simulink library "sensors_T2_design_lib"  (R2023b)
settings: Solver=ode45  StartTime=0.0  StopTime=10.0  RelTol=1e-3  EnableMultiTasking=on
undefined symbols (not defined in the file or in its folder): POS_hi, POS_lo, Timestep
libraries: NoiseModel_lib x16, simulink_extras x3, TransportDelay_lib x1, simulink x1
settings Model: Creator=amurch  LastModifiedBy=suvo
settings SolverCC: AlgebraicLoopSolver=TrustRegion
settings DataIOCC: LimitDataPoints=on  SaveFormat=Array  SignalLoggingSaveFormat=ModelDataLogs  ReturnWorkspaceOutputs=off
settings OptimizationCC: ExpressionDepthLimit=2147483647  LifeSpan=inf
settings DebuggingCC: UnderspecifiedInitializationDetection=Classic  MergeDetectMultiDrivingBlocksExec=none  SolverPrmCheckMsg=warning  FcnCallInpInsideContextMsg=warning  UnconnectedInputMsg=warning  UnconnectedOutputMsg=warning  UnconnectedLineMsg=warning  StateNameClashWarn=warning  SFUnexpectedBacktrackingDiag=warning  SFNoUnconditionalDefaultTransitionDiag=warning  SFExecutionAtInitializationDiag=none  ArithmeticOperatorsInVariantConditions=warning
settings HardwareCC: ProdBitPerPointer=32  ProdBitPerSizeT=32  ProdBitPerPtrDiffT=32  ProdLargestAtomicFloat=None  ProdIntDivRoundTo=Undefined  ProdEndianess=Unspecified  ProdWordSize=32  ProdHWDeviceType=32-bit Generic
settings ModelReferenceCC: PropagateSignalLabelsOutOfModel=off
settings SFSimCC: SimUseLocalCustomCode=off  CustomCodeUndefinedFunction=UseInterfaceOnly
settings RTWCC: RTWUseLocalCustomCode=off
settings CodeAppCC: StateflowObjectComments=on
settings GRTTargetCC: TargetLangStandard=C89/C90 (ANSI)  CombineOutputUpdateFcns=off  GRTInterface=on
settings ConfigComp: CovMetricSettings=dw  CovSaveCumulativeToWorkspaceVar=on  CovSaveSingleToWorkspaceVar=on

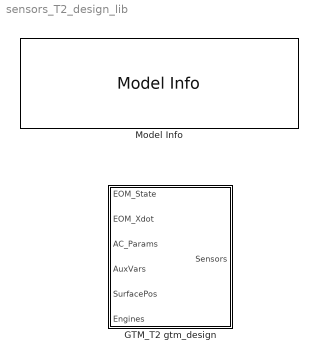
== system sensors_T2_design_lib ==
  GTM_T2 gtm_design : Subsystem
  Model Info : simulink/Model-Wide Utilities/Model Info  Frame=on  DisplayStringWithTags=|  HorizontalTextAlignment=Center  LeftAlignmentValue=0.5
      | Sensor Model Library
      | %<ModelVersion>
      | Las modified by %<LastModifiedBy> on %<LastModificationDate>

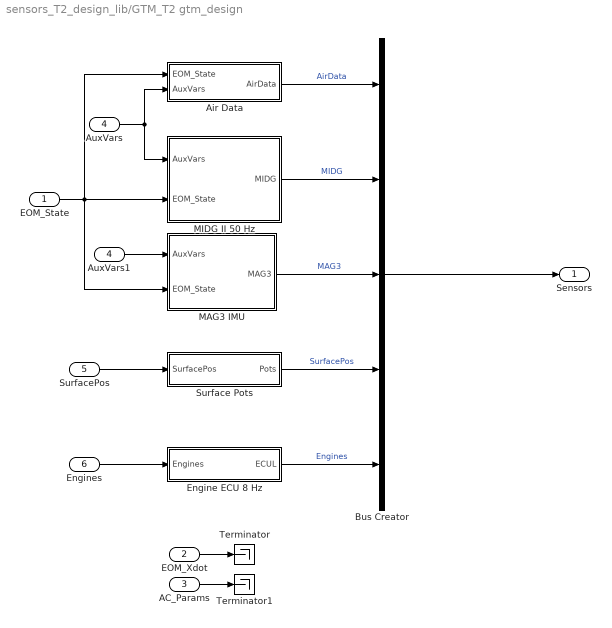
== system sensors_T2_design_lib/GTM_T2 gtm_design ==
  EOM_State : Inport
  EOM_Xdot : Inport  Port=2
  AC_Params : Inport  Port=3
  AuxVars : Inport  Port=4
  SurfacePos : Inport  Port=5
  Engines : Inport  Port=6
  Air Data : Subsystem
  AuxVars1 : InportShadow  Port=4
  Bus Creator : BusCreator  Inputs=5
  Engine ECU 8 Hz : Subsystem  SystemSampleTime=round(1/Timestep/8)*Timestep
  MAG3 IMU : Subsystem
  MIDG II 50 Hz : Subsystem  SystemSampleTime=round(1/Timestep/50)*Timestep
  Surface Pots : Subsystem
  Terminator : Terminator
  Terminator1 : Terminator
  Sensors : Outport
  wires:
  AuxVars1/1 -> MAG3 IMU/1(AuxVars)
  EOM_State/1 -> Air Data/1(EOM_State), MIDG II 50 Hz/2(EOM_State), MAG3 IMU/2(EOM_State)
  AuxVars/1 -> MIDG II 50 Hz/1(AuxVars), Air Data/2(AuxVars)
  SurfacePos/1 -> Surface Pots/1(SurfacePos)
  Engines/1 -> Engine ECU 8 Hz/1(Engines)
  MAG3 IMU/1(MAG3) -> Bus Creator/3  "MAG3"
  Engine ECU 8 Hz/1(ECUL) -> Bus Creator/5  "Engines"
  Surface Pots/1(Pots) -> Bus Creator/4  "SurfacePos"
  MIDG II 50 Hz/1(MIDG) -> Bus Creator/2  "MIDG"
  Air Data/1(AirData) -> Bus Creator/1  "AirData"
  Bus Creator/1 -> Sensors/1
  EOM_Xdot/1 -> Terminator/1
  AC_Params/1 -> Terminator1/1

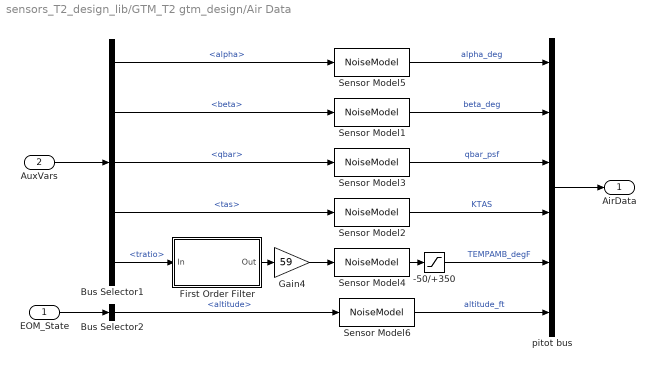
== system sensors_T2_design_lib/GTM_T2 gtm_design/Air Data ==
  EOM_State : Inport
  AuxVars : Inport  Port=2
  -50/+350 : Saturate  UpperLimit=350  LowerLimit=-50
  Bus Selector1 : BusSelector  OutputSignals=alpha,beta,qbar,tas,tratio
  Bus Selector2 : BusSelector  OutputSignals=altitude
  First Order Filter : Subsystem  mask(first order filter){tau=6}
      mask help:
      | __1__
      |  tau s+1
      |
      | First order filter  transfer function
      | with integrator IC = input  at time=0
      | If tau < Simulation Timestep, input is passed through unchanged
      | Simulation timestep must be a variable in the model/base workspace named
      | "Timestep"
      mask Help:
      | This block models a first order filter with the initial condition
      | on the integrator set to the steady state value for constant input.
      | time constant is an input
      mask Display: fprintf('  1\n--------------\n %2.1g s + 1', tau)
  Gain4 : Gain  Gain=59
  Sensor Model1 : NoiseModel_lib/NoiseModel  SystemSampleTime=-1  noise_on=SensorNoise.On  sigma=SensorNoise.beta.Std  seed=878224  bias=SensorNoise.beta.Bias  scf=SensorNoise.beta.Scf
  Sensor Model2 : NoiseModel_lib/NoiseModel  SystemSampleTime=-1  noise_on=SensorNoise.On  sigma=SensorNoise.KTAS.Std  seed=878654  bias=SensorNoise.KTAS.Bias  scf=SensorNoise.KTAS.Scf
  Sensor Model3 : NoiseModel_lib/NoiseModel  SystemSampleTime=-1  noise_on=SensorNoise.On  sigma=SensorNoise.dyn_press.Std  seed=848234  bias=SensorNoise.dyn_press.Bias  scf=SensorNoise.dyn_press.Scf
  Sensor Model4 : NoiseModel_lib/NoiseModel  SystemSampleTime=-1  noise_on=SensorNoise.On  sigma=SensorNoise.tempamb.Std  seed=878634  bias=SensorNoise.tempamb.Bias  scf=SensorNoise.tempamb.Scf
  Sensor Model5 : NoiseModel_lib/NoiseModel  SystemSampleTime=-1  noise_on=SensorNoise.On  sigma=SensorNoise.alpha.Std  seed=278234  bias=SensorNoise.alpha.Bias  scf=SensorNoise.alpha.Scf
  Sensor Model6 : NoiseModel_lib/NoiseModel  SystemSampleTime=-1  noise_on=SensorNoise.On  sigma=SensorNoise.baro_alt.Std  seed=878654  bias=SensorNoise.baro_alt.Bias  scf=SensorNoise.baro_alt.Scf
  pitot bus : BusCreator  Inputs=6
  AirData : Outport
  wires:
  EOM_State/1 -> Bus Selector2/1
  Sensor Model6/1 -> pitot bus/6  "altitude_ft"
  Bus Selector2/1 -> Sensor Model6/1  "<altitude>"
  AuxVars/1 -> Bus Selector1/1
  Sensor Model2/1 -> pitot bus/4  "KTAS"
  Bus Selector1/4 -> Sensor Model2/1  "<tas>"
  Sensor Model1/1 -> pitot bus/2  "beta_deg"
  Sensor Model5/1 -> pitot bus/1  "alpha_deg"
  Bus Selector1/2 -> Sensor Model1/1  "<beta>"
  Bus Selector1/1 -> Sensor Model5/1  "<alpha>"
  First Order Filter/1(Out) -> Gain4/1
  -50/+350/1 -> pitot bus/5  "TEMPAMB_degF"
  Sensor Model4/1 -> -50/+350/1
  Gain4/1 -> Sensor Model4/1
  pitot bus/1 -> AirData/1
  Bus Selector1/3 -> Sensor Model3/1  "<qbar>"
  Sensor Model3/1 -> pitot bus/3  "qbar_psf"
  Bus Selector1/5 -> First Order Filter/1(In)  "<tratio>"

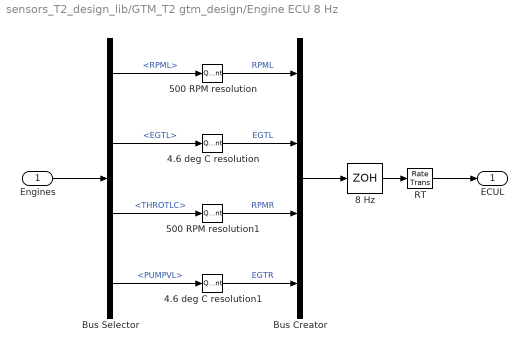
== system sensors_T2_design_lib/GTM_T2 gtm_design/Engine ECU 8 Hz ==
  Engines : Inport
  4.6 deg C resolution : Quantizer  QuantizationInterval=4.6
  4.6 deg C resolution1 : Quantizer  QuantizationInterval=4.6
  500 RPM resolution : Quantizer  QuantizationInterval=500
  500 RPM resolution1 : Quantizer  QuantizationInterval=500
  8 Hz : ZeroOrderHold  SampleTime=round(1/Timestep/8)*Timestep
  Bus Creator : BusCreator  Inputs=4
  Bus Selector : BusSelector  OutputSignals=RPML,EGTL,THROTLC,PUMPVL
  RT : RateTransition
  ECUL : Outport
  wires:
  4.6 deg C resolution1/1 -> Bus Creator/4  "EGTR"
  Bus Selector/4 -> 4.6 deg C resolution1/1  "<PUMPVL>"
  500 RPM resolution1/1 -> Bus Creator/3  "RPMR"
  Bus Selector/3 -> 500 RPM resolution1/1  "<THROTLC>"
  Engines/1 -> Bus Selector/1
  4.6 deg C resolution/1 -> Bus Creator/2  "EGTL"
  500 RPM resolution/1 -> Bus Creator/1  "RPML"
  Bus Selector/1 -> 500 RPM resolution/1  "<RPML>"
  RT/1 -> ECUL/1
  Bus Creator/1 -> 8 Hz/1
  8 Hz/1 -> RT/1
  Bus Selector/2 -> 4.6 deg C resolution/1  "<EGTL>"

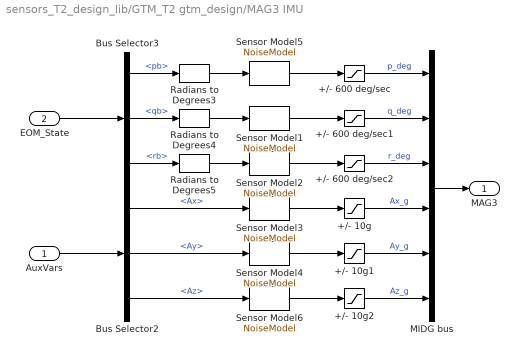
== system sensors_T2_design_lib/GTM_T2 gtm_design/MAG3 IMU ==
  AuxVars : Inport
  EOM_State : Inport  Port=2
  +/- 10g : Saturate  UpperLimit=10  LowerLimit=-10
  +/- 10g1 : Saturate  UpperLimit=10  LowerLimit=-10
  +/- 10g2 : Saturate  UpperLimit=10  LowerLimit=-10
  +/- 600 deg/sec : Saturate  UpperLimit=600  LowerLimit=-600
  +/- 600 deg/sec1 : Saturate  UpperLimit=600  LowerLimit=-600
  +/- 600 deg/sec2 : Saturate  UpperLimit=600  LowerLimit=-600
  Bus Selector2 : BusSelector  OutputSignals=Ax,Ay,Az
  Bus Selector3 : BusSelector  OutputSignals=pb,qb,rb
  MIDG bus : BusCreator  Inputs=6
  Radians to Degrees3 : simulink_extras/Transformations/Radians to Degrees  SystemSampleTime=-1
  Radians to Degrees4 : simulink_extras/Transformations/Radians to Degrees  SystemSampleTime=-1
  Radians to Degrees5 : simulink_extras/Transformations/Radians to Degrees  SystemSampleTime=-1
  Sensor Model1 : NoiseModel_lib/NoiseModel  SystemSampleTime=-1  noise_on=SensorNoise.On  sigma=SensorNoise.MAG3.qdeg.Std  seed=871234  bias=SensorNoise.MAG3.qdeg.Bias  scf=SensorNoise.MAG3.qdeg.Scf
  Sensor Model2 : NoiseModel_lib/NoiseModel  SystemSampleTime=-1  noise_on=SensorNoise.On  sigma=SensorNoise.MAG3.rdeg.Std  seed=878134  bias=SensorNoise.MAG3.rdeg.Bias  scf=SensorNoise.MAG3.rdeg.Scf
  Sensor Model3 : NoiseModel_lib/NoiseModel  SystemSampleTime=-1  noise_on=SensorNoise.On  sigma=SensorNoise.MAG3.nxbody.Std  seed=878234  bias=SensorNoise.MAG3.nxbody.Bias  scf=SensorNoise.MAG3.nxbody.Scf
  Sensor Model4 : NoiseModel_lib/NoiseModel  SystemSampleTime=-1  noise_on=SensorNoise.On  sigma=SensorNoise.MAG3.nybody.Std  seed=8782345  bias=SensorNoise.MAG3.nybody.Bias  scf=SensorNoise.MAG3.nybody.Scf
  Sensor Model5 : NoiseModel_lib/NoiseModel  SystemSampleTime=-1  noise_on=SensorNoise.On  sigma=SensorNoise.MAG3.pdeg.Std  seed=878233  bias=SensorNoise.MAG3.pdeg.Bias  scf=SensorNoise.MAG3.pdeg.Scf
  Sensor Model6 : NoiseModel_lib/NoiseModel  SystemSampleTime=-1  noise_on=SensorNoise.On  sigma=SensorNoise.MAG3.nzbody.Std  seed=878236  bias=SensorNoise.MAG3.nzbody.Bias  scf=SensorNoise.MAG3.nzbody.Scf
  MAG3 : Outport
  wires:
  MIDG bus/1 -> MAG3/1
  AuxVars/1 -> Bus Selector2/1
  Sensor Model5/1 -> +/- 600 deg/sec/1
  Sensor Model6/1 -> +/- 10g2/1
  Sensor Model4/1 -> +/- 10g1/1
  Sensor Model3/1 -> +/- 10g/1
  Sensor Model2/1 -> +/- 600 deg/sec2/1
  Sensor Model1/1 -> +/- 600 deg/sec1/1
  Radians to Degrees5/1 -> Sensor Model2/1
  Radians to Degrees4/1 -> Sensor Model1/1
  Radians to Degrees3/1 -> Sensor Model5/1
  Bus Selector2/3 -> Sensor Model6/1  "<Az>"
  Bus Selector2/2 -> Sensor Model4/1  "<Ay>"
  Bus Selector2/1 -> Sensor Model3/1  "<Ax>"
  Bus Selector3/3 -> Radians to Degrees5/1  "<rb>"
  Bus Selector3/2 -> Radians to Degrees4/1  "<qb>"
  Bus Selector3/1 -> Radians to Degrees3/1  "<pb>"
  EOM_State/1 -> Bus Selector3/1
  +/- 600 deg/sec/1 -> MIDG bus/1  "p_deg"
  +/- 600 deg/sec1/1 -> MIDG bus/2  "q_deg"
  +/- 600 deg/sec2/1 -> MIDG bus/3  "r_deg"
  +/- 10g/1 -> MIDG bus/4  "Ax_g"
  +/- 10g1/1 -> MIDG bus/5  "Ay_g"
  +/- 10g2/1 -> MIDG bus/6  "Az_g"

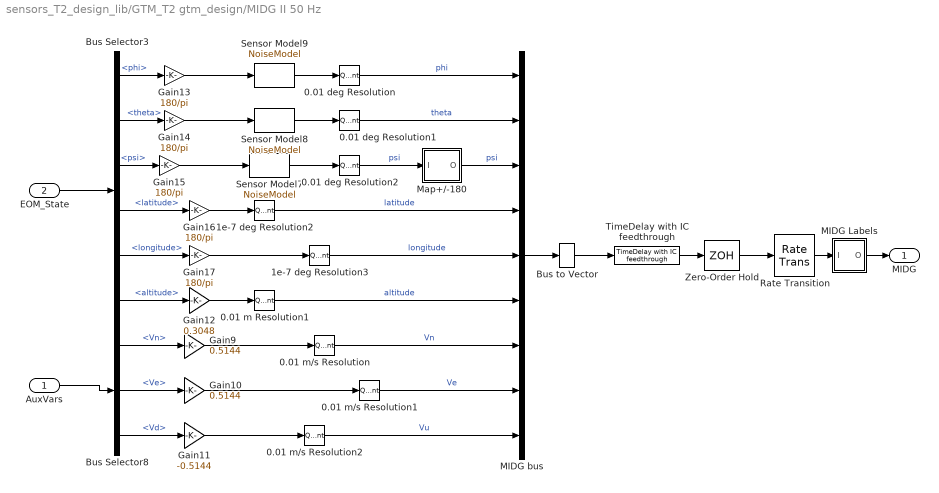
== system sensors_T2_design_lib/GTM_T2 gtm_design/MIDG II 50 Hz ==
  AuxVars : Inport
  EOM_State : Inport  Port=2
  0.01 deg Resolution : Quantizer  QuantizationInterval=0.01
  0.01 deg Resolution1 : Quantizer  QuantizationInterval=0.01
  0.01 deg Resolution2 : Quantizer  QuantizationInterval=0.01
  0.01 m Resolution1 : Quantizer  QuantizationInterval=0.01
  0.01 m/s Resolution : Quantizer  QuantizationInterval=0.01
  0.01 m/s Resolution1 : Quantizer  QuantizationInterval=0.01
  0.01 m/s Resolution2 : Quantizer  QuantizationInterval=0.01
  1e-7 deg Resolution2 : Quantizer  QuantizationInterval=1e-7
  1e-7 deg Resolution3 : Quantizer  QuantizationInterval=1e-7
  Bus Selector3 : BusSelector  OutputSignals=phi,theta,psi,latitude,longitude,altitude
  Bus Selector8 : BusSelector  OutputSignals=Vn,Ve,Vd
  Bus to Vector : BusToVector
  Gain10 : Gain  Gain=0.5144
  Gain11 : Gain  Gain=-0.5144
  Gain12 : Gain  Gain=0.3048
  Gain{13..17} (5 alike) : Gain  Gain=180/pi
  Gain9 : Gain  Gain=0.5144
  MIDG Labels : Subsystem
  MIDG bus : BusCreator  Inputs=9
  Map+/-180 : Subsystem
  Rate Transition : RateTransition
  Sensor Model7 : NoiseModel_lib/NoiseModel  SystemSampleTime=-1  noise_on=SensorNoise.On  sigma=SensorNoise.MIDG.psi.Std  seed=878232  bias=SensorNoise.MIDG.psi.Bias  scf=SensorNoise.MIDG.psi.Scf
  Sensor Model8 : NoiseModel_lib/NoiseModel  SystemSampleTime=-1  noise_on=SensorNoise.On  sigma=SensorNoise.MIDG.theta.Std  seed=878231  bias=SensorNoise.MIDG.theta.Bias  scf=SensorNoise.MIDG.theta.Scf
  Sensor Model9 : NoiseModel_lib/NoiseModel  SystemSampleTime=-1  noise_on=SensorNoise.On  sigma=SensorNoise.MIDG.phi.Std  seed=878230  bias=SensorNoise.MIDG.phi.Bias  scf=SensorNoise.MIDG.phi.Scf
  TimeDelay with IC feedthrough : TransportDelay_lib/TimeDelay with  IC feedthrough  SystemSampleTime=-1  TimeDelay=40e-3
  Zero-Order Hold : ZeroOrderHold  SampleTime=round(1/Timestep/50)*Timestep
  MIDG : Outport
  wires:
  Rate Transition/1 -> MIDG Labels/1(I)
  0.01 m/s Resolution2/1 -> MIDG bus/9  "Vu"
  MIDG Labels/1(O) -> MIDG/1
  Map+/-180/1(O) -> MIDG bus/3  "psi"
  AuxVars/1 -> Bus Selector8/1
  Bus Selector3/6 -> Gain12/1  "<altitude>"
  Bus Selector3/5 -> Gain17/1  "<longitude>"
  Bus Selector3/4 -> Gain16/1  "<latitude>"
  Bus Selector8/3 -> Gain11/1  "<Vd>"
  Bus Selector8/2 -> Gain10/1  "<Ve>"
  Bus Selector8/1 -> Gain9/1  "<Vn>"
  Gain17/1 -> 1e-7 deg Resolution3/1
  Gain16/1 -> 1e-7 deg Resolution2/1
  Gain15/1 -> Sensor Model7/1
  Gain14/1 -> Sensor Model8/1
  Gain13/1 -> Sensor Model9/1
  0.01 m/s Resolution1/1 -> MIDG bus/8  "Ve"
  0.01 m/s Resolution/1 -> MIDG bus/7  "Vn"
  Gain12/1 -> 0.01 m Resolution1/1
  Gain11/1 -> 0.01 m/s Resolution2/1
  Gain10/1 -> 0.01 m/s Resolution1/1
  Gain9/1 -> 0.01 m/s Resolution/1
  0.01 m Resolution1/1 -> MIDG bus/6  "altitude"
  1e-7 deg Resolution3/1 -> MIDG bus/5  "longitude"
  1e-7 deg Resolution2/1 -> MIDG bus/4  "latitude"
  0.01 deg Resolution2/1 -> Map+/-180/1(I)  "psi"
  0.01 deg Resolution1/1 -> MIDG bus/2  "theta"
  0.01 deg Resolution/1 -> MIDG bus/1  "phi"
  Sensor Model9/1 -> 0.01 deg Resolution/1
  Sensor Model8/1 -> 0.01 deg Resolution1/1
  Sensor Model7/1 -> 0.01 deg Resolution2/1
  Bus Selector3/3 -> Gain15/1  "<psi>"
  Bus Selector3/2 -> Gain14/1  "<theta>"
  Bus Selector3/1 -> Gain13/1  "<phi>"
  EOM_State/1 -> Bus Selector3/1
  Zero-Order Hold/1 -> Rate Transition/1
  MIDG bus/1 -> Bus to Vector/1
  TimeDelay with IC feedthrough/1 -> Zero-Order Hold/1
  Bus to Vector/1 -> TimeDelay with IC feedthrough/1

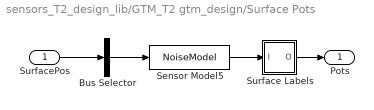
== system sensors_T2_design_lib/GTM_T2 gtm_design/Surface Pots ==
  SurfacePos : Inport
  Bus Selector : BusSelector  OutputSignals=ELLOB,ELLIB,ELROB,ELRIB,AILL,AILR,RUDU,RUDL,FLAPLIB,FLAPLOB,FLAPRIB,FLAPROB  OutputAsBus=on
  Sensor Model5 : NoiseModel_lib/NoiseModel  SystemSampleTime=-1  noise_on=SensorNoise.On  sigma=SensorNoise.pots.Std  seed=878239  bias=SensorNoise.pots.Bias  scf=SensorNoise.pots.Scf
  Surface Labels : Subsystem
  Pots : Outport
  wires:
  Surface Labels/1(O) -> Pots/1
  Sensor Model5/1 -> Surface Labels/1(I)
  SurfacePos/1 -> Bus Selector/1
  Bus Selector/1 -> Sensor Model5/1

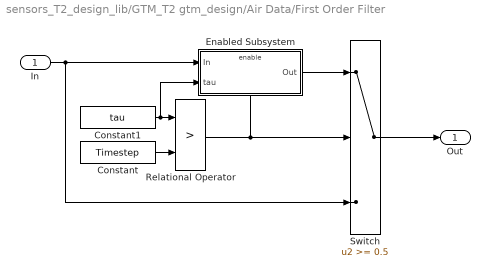
== system sensors_T2_design_lib/GTM_T2 gtm_design/Air Data/First Order Filter ==
  In : Inport
  Constant : Constant  Value=Timestep
  Constant1 : Constant  Value=tau
  Enabled Subsystem : Subsystem  TreatAsAtomicUnit=on
  Relational Operator : RelationalOperator  Operator=>  OutDataTypeStr=boolean  InputSameDT=off
  Switch : Switch  Threshold=0.5  SaturateOnIntegerOverflow=off  InputSameDT=off
  Out : Outport
  wires:
  Constant/1 -> Relational Operator/2
  Relational Operator/1 -> Switch/2, Enabled Subsystem/Enable
  In/1 -> Switch/3, Enabled Subsystem/1(In)
  Switch/1 -> Out/1
  Enabled Subsystem/1(Out) -> Switch/1
  Constant1/1 -> Relational Operator/1, Enabled Subsystem/2(tau)

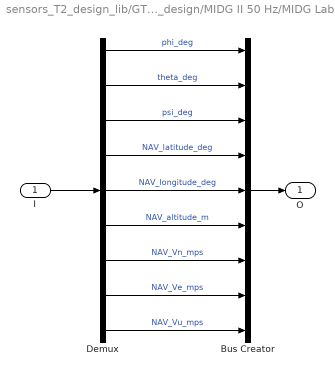
== system sensors_T2_design_lib/GTM_T2 gtm_design/MIDG II 50 Hz/MIDG Labels ==
  I : Inport
  Bus Creator : BusCreator  Inputs=9
  Demux : Demux  Outputs=9
  O : Outport
  wires:
  Demux/9 -> Bus Creator/9  "NAV_Vu_mps"
  Demux/8 -> Bus Creator/8  "NAV_Ve_mps"
  Demux/7 -> Bus Creator/7  "NAV_Vn_mps"
  Demux/6 -> Bus Creator/6  "NAV_altitude_m"
  Demux/5 -> Bus Creator/5  "NAV_longitude_deg"
  Demux/4 -> Bus Creator/4  "NAV_latitude_deg"
  Demux/1 -> Bus Creator/1  "phi_deg"
  Demux/3 -> Bus Creator/3  "psi_deg"
  Demux/2 -> Bus Creator/2  "theta_deg"
  Bus Creator/1 -> O/1
  I/1 -> Demux/1

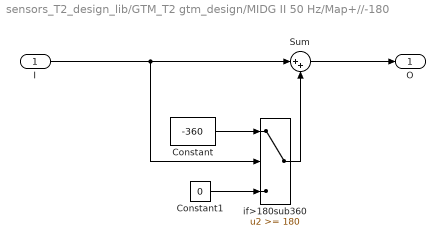
== system sensors_T2_design_lib/GTM_T2 gtm_design/MIDG II 50 Hz/Map+//-180 ==
  I : Inport
  Constant : Constant  Value=-360
  Constant1 : Constant  Value=0
  Sum : Sum  Inputs=|++
  if>180sub360 : Switch  Threshold=180  SaturateOnIntegerOverflow=off  InputSameDT=off
  O : Outport
  wires:
  Constant/1 -> if>180sub360/1
  Constant1/1 -> if>180sub360/3
  I/1 -> Sum/1, if>180sub360/2
  Sum/1 -> O/1
  if>180sub360/1 -> Sum/2

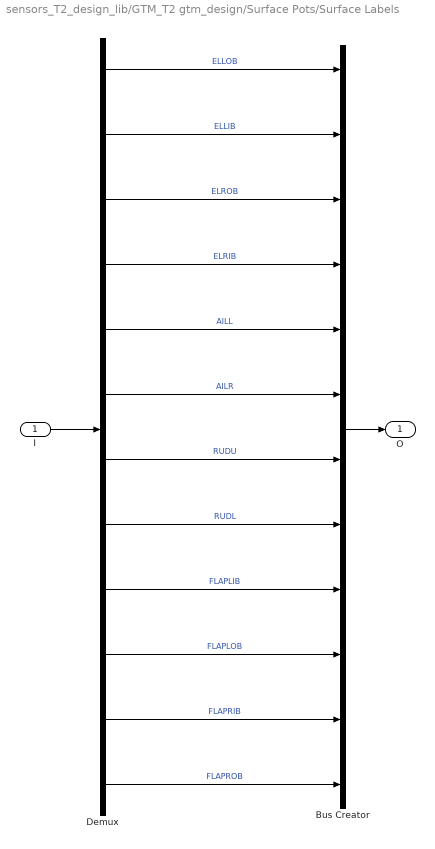
== system sensors_T2_design_lib/GTM_T2 gtm_design/Surface Pots/Surface Labels ==
  I : Inport
  Bus Creator : BusCreator  Inputs=12
  Demux : Demux  Outputs=12
  O : Outport
  wires:
  I/1 -> Demux/1
  Demux/1 -> Bus Creator/1  "ELLOB"
  Demux/2 -> Bus Creator/2  "ELLIB"
  Demux/3 -> Bus Creator/3  "ELROB"
  Demux/4 -> Bus Creator/4  "ELRIB"
  Demux/5 -> Bus Creator/5  "AILL"
  Demux/6 -> Bus Creator/6  "AILR"
  Demux/7 -> Bus Creator/7  "RUDU"
  Demux/8 -> Bus Creator/8  "RUDL"
  Demux/9 -> Bus Creator/9  "FLAPLIB"
  Demux/10 -> Bus Creator/10  "FLAPLOB"
  Demux/11 -> Bus Creator/11  "FLAPRIB"
  Demux/12 -> Bus Creator/12  "FLAPROB"
  Bus Creator/1 -> O/1

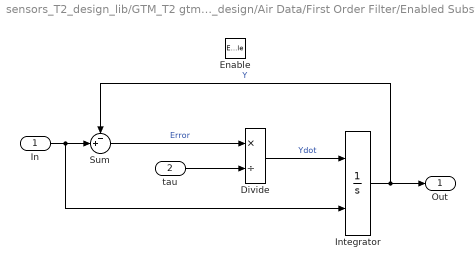
== system sensors_T2_design_lib/GTM_T2 gtm_design/Air Data/First Order Filter/Enabled Subsystem ==
  In : Inport
  tau : Inport  Port=2
  Enable : EnablePort
  Divide : Product  Inputs=*/
  Integrator : Integrator  InitialConditionSource=external  UpperSaturationLimit=POS_hi  LowerSaturationLimit=POS_lo
  Sum : Sum  Inputs=-+|  InputSameDT=on  SaturateOnIntegerOverflow=on  OutDataTypeStr=Inherit: Same as first input
  Out : Outport
  wires:
  Divide/1 -> Integrator/1  "Ydot"
  tau/1 -> Divide/2
  Integrator/1 -> Sum/1, Out/1  "Y"
  In/1 -> Integrator/2, Sum/2
  Sum/1 -> Divide/1  "Error"
